simulink model "linetap2"  (Simulink 8.5)
settings: Solver=ode15s  SolverMode=SingleTasking  StartTime=0.0  StopTime=0.1  RelTol=1e-3  AbsTol=1e-3
libraries: powerlib x37
settings Model: Creator=Dr. Lotfifard  LastModifiedBy=PC
settings DataIOCC: LimitDataPoints=off
settings OptimizationCC: BlockReduction=off  BooleanDataType=off
settings DebuggingCC: SaveWithParameterizedLinksMsg=none  SignalResolutionControl=TryResolveAllWithWarning  MultiTaskDSMMsg=warning  MultiTaskCondExecSysMsg=none  FcnCallInpInsideContextMsg=UseLocalSettings  StrictBusMsg=None
settings HardwareCC: TargetUnknown=on

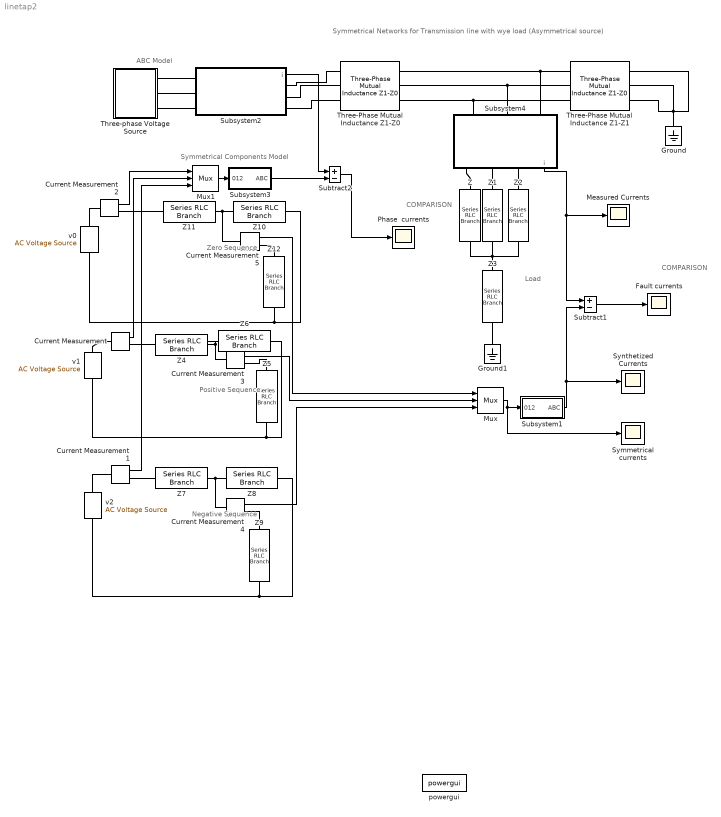
== system linetap2 ==
  note: Symmetrical Networks for Transmission line with wye load (Asymmetrical source)
  note: ABC Model
  note: Symmetrical Components Model
  note: Load
  note: Zero
      | Sequence
  note: Positive
      | Sequence
  note: Negative
      | Sequence
  note: COMPARISON
  note: COMPARISON
  Current Measurement : powerlib/Measurements/Current Measurement  Tag=PoWeRsYsTeMmEaSuReMeNtFiRsT  PhasorSimulation=off  OutputType=Complex  PSBequivalent=0
  Current Measurement{1..5} (5 alike) : powerlib/Measurements/Current Measurement  Tag=PoWeRsYsTeMmEaSuReMeNt  PhasorSimulation=off  OutputType=Complex  PSBequivalent=0
  Fault currents : Scope
      settings: TickLabels=on  TimeRange=0.1  YMin=-3  YMax=3
  Ground : powerlib/Elements/Ground  LConnTagsString=a
  Ground1 : powerlib/Elements/Ground  LConnTagsString=a
  Measured Currents : Scope
      settings: TickLabels=on  TimeRange=0.1  YMin=-3  YMax=3  SaveName=ScopeData2
  Mux : Mux  Inputs=3
  Mux1 : Mux  Inputs=3
  Phase  currents : Scope
      settings: TickLabels=on  TimeRange=0.1  YMin=-23  YMax=23  SaveName=ScopeData3
  Subsystem1 : Subsystem
  Subsystem2 : Subsystem
      mask Display: disp('Current\nMeasurements')
  Subsystem3 : Subsystem
  Subsystem4 : Subsystem
      mask Display: disp('Current\nMeasurements')
  Subtract1 : Sum  Inputs=+-  SaturateOnIntegerOverflow=on  InputSameDT=on  OutDataTypeStr=Inherit: Same as first input
  Subtract2 : Sum  Inputs=+-  SaturateOnIntegerOverflow=on  InputSameDT=on  OutDataTypeStr=Inherit: Same as first input
  Symmetrical currents : Scope
      settings: TickLabels=on  TimeRange=0.05  YMin=-1.05  YMax=1.05  SaveName=ScopeData4
  Synthetized Currents : Scope
      settings: TickLabels=on  TimeRange=0.1  YMin=-3  YMax=3
  Three-Phase Mutual Inductance Z1-Z0 : powerlib/Elements/Three-Phase Mutual Inductance Z1-Z0  LConnTagsString=a|b|c  RConnTagsString=A|B|C  PositiveSequence="[ 0.003  0.015/(2*pi*60)]"  ZeroSequence="[0.006  0.03/(2*pi*60)]"
  Three-Phase Mutual Inductance Z1-Z1 : powerlib/Elements/Three-Phase Mutual Inductance Z1-Z0  LConnTagsString=a|b|c  RConnTagsString=A|B|C  PositiveSequence="[ 0.007  0.035/(2*pi*60)]"  ZeroSequence="[ 0.014  0.07/(2*pi*60)]"
  Three-phase Voltage Source : Subsystem
  Z{,1..2,5,9,12} (6 alike) : powerlib/Elements/Series RLC Branch  LConnTagsString=__new0  RConnTagsString=__new0  BranchType=RL  Resistance=0.72  Inductance=0.54/(2*pi*60)  SetiL0=off  InitialCurrent=0  Capacitance=1e-6  Setx0=off  InitialVoltage=0  Measurements=None
  Z10 : powerlib/Elements/Series RLC Branch  LConnTagsString=__new0  RConnTagsString=__new0  BranchType=RL  Resistance=0.014  Inductance=0.07/(2*pi*60)  SetiL0=off  InitialCurrent=0  Capacitance=1e-6  Setx0=off  InitialVoltage=0  Measurements=None
  Z11 : powerlib/Elements/Series RLC Branch  LConnTagsString=__new0  RConnTagsString=__new0  BranchType=RL  Resistance=0.006  Inductance=0.03/(2*pi*60)  SetiL0=off  InitialCurrent=0  Capacitance=1e-6  Setx0=off  InitialVoltage=0  Measurements=None
  Z3 : powerlib/Elements/Series RLC Branch  LConnTagsString=__new0  RConnTagsString=__new0  BranchType=RL  Resistance=1  Inductance=0  SetiL0=off  InitialCurrent=0  Capacitance=1e-6  Setx0=off  InitialVoltage=0  Measurements=None
  Z4 : powerlib/Elements/Series RLC Branch  LConnTagsString=__new0  RConnTagsString=__new0  BranchType=RL  Resistance=0.003  Inductance=0.015/(2*pi*60)  SetiL0=off  InitialCurrent=0  Capacitance=1e-6  Setx0=off  InitialVoltage=0  Measurements=None
  Z6 : powerlib/Elements/Series RLC Branch  LConnTagsString=__new0  RConnTagsString=__new0  BranchType=RL  Resistance=0.007  Inductance=0.035/(2*pi*60)  SetiL0=off  InitialCurrent=0  Capacitance=1e-6  Setx0=off  InitialVoltage=0  Measurements=None
  Z7 : powerlib/Elements/Series RLC Branch  LConnTagsString=__new0  RConnTagsString=__new0  BranchType=RL  Resistance=0.003  Inductance=0.015/(2*pi*60)  SetiL0=off  InitialCurrent=0  Capacitance=1e-6  Setx0=off  InitialVoltage=0  Measurements=None
  Z8 : powerlib/Elements/Series RLC Branch  LConnTagsString=__new0  RConnTagsString=__new0  BranchType=RL  Resistance=0.007  Inductance=0.035/(2*pi*60)  SetiL0=off  InitialCurrent=0  Capacitance=1e-6  Setx0=off  InitialVoltage=0  Measurements=None
  powergui : powerlib/powergui  SimulationMode=Continuous  SolverType=Tustin/Backward Euler (TBE)  SampleTime=0  frequency=60  SPID=off  DisableSnubberDevices=off  DisableRonSwitches=off  DisableVfSwitches=off  SwTol=0  DisplayEquations=off  Interpol=off  methode=off  Ts=0  FunctionMessages=off  echomessages=off  HookPort=off  EnableUseOfTLC=off  x0status=blocks  frequencyindice=60  Pbase=100e6  ErrMax=1e-4  Iterations=50  UnitsV=kV  UnitsW=MW  buscounter=0  RestoreLinks=warning  ResistiveCurrentMeasurement=off  Frange=[0:2:500]  Ylog=off  Xlog=on  ShowGrid=off  save=off  variable=ZData  structure=0  ZoomFFT=on  StartTime=0.0  cycles=1  DisplayStyle=1  fundamental=60  FreqAxis=off  MaxFrequency=1000  frequencyindicesteady=1  RmsSteady=1  display=off
  v0 : powerlib/Electrical Sources/AC Voltage Source  Amplitude=0.031  Phase=-78  Frequency=60  SampleTime=0  Measurements=None
  v1 : powerlib/Electrical Sources/AC Voltage Source  Amplitude=0.963  Phase=-6.56  Frequency=60  SampleTime=0  Measurements=None
  v2 : powerlib/Electrical Sources/AC Voltage Source  Amplitude=0.145  Phase=75.41  Frequency=60  SampleTime=0  Measurements=None
  wires:
  Mux/1 -> Symmetrical currents/1, Subsystem1/1(012)
  Mux1/1 -> Subsystem3/1(012)
  Current Measurement/1 -> Mux1/2
  Subtract2/1 -> Phase  currents/1
  Current Measurement4/1 -> Mux/3
  Current Measurement3/1 -> Mux/2
  Current Measurement1/1 -> Mux1/3
  Current Measurement2/1 -> Mux1/1
  Current Measurement5/1 -> Mux/1
  Subtract1/1 -> Fault currents/1
  Subsystem1/1(ABC) -> Subtract1/2, Synthetized Currents/1
  Subsystem3/1(ABC) -> Subtract2/2
  Subsystem4/1(i) -> Measured Currents/1, Subtract1/1
  Subsystem2/1(i) -> Subtract2/1
  connections:
  Three-Phase Mutual Inductance Z1-Z1/RConn3 -- Three-Phase Mutual Inductance Z1-Z1/RConn2 -- Ground/LConn1 -- Three-Phase Mutual Inductance Z1-Z1/RConn1
  Z/RConn1 -- Z1/RConn1 -- Z3/LConn1 -- Z2/RConn1
  Subsystem4/LConn1 -- Three-Phase Mutual Inductance Z1-Z0/RConn1 -- Three-Phase Mutual Inductance Z1-Z1/LConn1
  Subsystem4/LConn2 -- Three-Phase Mutual Inductance Z1-Z0/RConn2 -- Three-Phase Mutual Inductance Z1-Z1/LConn2
  Subsystem4/LConn3 -- Three-Phase Mutual Inductance Z1-Z0/RConn3 -- Three-Phase Mutual Inductance Z1-Z1/LConn3
  Z6/LConn1 -- Current Measurement3/LConn1 -- Z4/RConn1
  Z6/RConn1 -- Z5/RConn1 -- v1/LConn1
  Z8/LConn1 -- Z7/RConn1 -- Current Measurement4/LConn1
  v2/LConn1 -- Z8/RConn1 -- Z9/RConn1
  Current Measurement5/LConn1 -- Z10/LConn1 -- Z11/RConn1
  v0/LConn1 -- Z10/RConn1 -- Z12/RConn1
  Z/LConn1 -- Subsystem4/RConn3
  Z2/LConn1 -- Subsystem4/RConn1
  Z1/LConn1 -- Subsystem4/RConn2
  Current Measurement5/RConn1 -- Z12/LConn1
  Current Measurement/RConn1 -- Z4/LConn1
  Z5/LConn1 -- Current Measurement3/RConn1
  Subsystem2/RConn1 -- Three-Phase Mutual Inductance Z1-Z0/LConn1
  Z11/LConn1 -- Current Measurement2/RConn1
  Subsystem2/LConn3 -- Three-phase Voltage Source/RConn3
  Subsystem2/LConn1 -- Three-phase Voltage Source/RConn1
  Three-phase Voltage Source/RConn2 -- Subsystem2/LConn2
  Z3/RConn1 -- Ground1/LConn1
  Current Measurement4/RConn1 -- Z9/LConn1
  Current Measurement2/LConn1 -- v0/RConn1
  Z7/LConn1 -- Current Measurement1/RConn1
  Current Measurement/LConn1 -- v1/RConn1
  Three-Phase Mutual Inductance Z1-Z0/LConn2 -- Subsystem2/RConn2
  Subsystem2/RConn3 -- Three-Phase Mutual Inductance Z1-Z0/LConn3
  Current Measurement1/LConn1 -- v2/RConn1

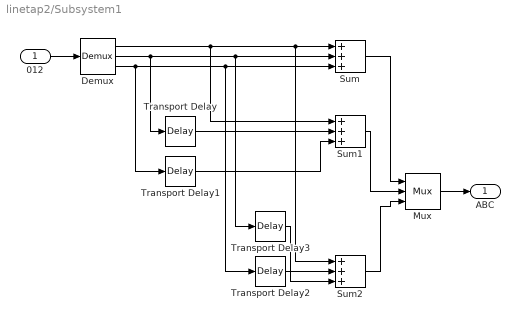
== system linetap2/Subsystem1 ==
  012 : Inport
  Demux : Demux  Outputs=3
  Mux : Mux  Inputs=3
  Sum : Sum  Inputs=+++  SaturateOnIntegerOverflow=on  InputSameDT=on  OutDataTypeStr=Inherit: Same as first input
  Sum1 : Sum  Inputs=+++  SaturateOnIntegerOverflow=on  InputSameDT=on  OutDataTypeStr=Inherit: Same as first input
  Sum2 : Sum  Inputs=+++  SaturateOnIntegerOverflow=on  InputSameDT=on  OutDataTypeStr=Inherit: Same as first input
  Transport Delay : TransportDelay  DelayTime=1/(3*60)
  Transport Delay1 : TransportDelay  DelayTime=2/(3*60)
  Transport Delay2 : TransportDelay  DelayTime=1/(3*60)
  Transport Delay3 : TransportDelay  DelayTime=2/(3*60)
  ABC : Outport  InitialOutput=0
  wires:
  Transport Delay3/1 -> Sum2/2
  Transport Delay2/1 -> Sum2/3
  Transport Delay1/1 -> Sum1/3
  Transport Delay/1 -> Sum1/2
  Demux/1 -> Sum2/1, Sum/1, Sum1/1
  Demux/3 -> Transport Delay2/1, Sum/3, Transport Delay1/1
  Demux/2 -> Transport Delay3/1, Sum/2, Transport Delay/1
  Sum2/1 -> Mux/3
  Mux/1 -> ABC/1
  Sum/1 -> Mux/1
  Sum1/1 -> Mux/2
  012/1 -> Demux/1

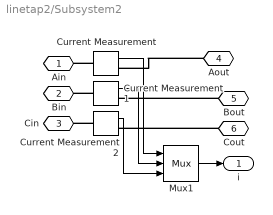
== system linetap2/Subsystem2 ==
  Current Measurement : powerlib/Measurements/Current Measurement  Tag=PoWeRsYsTeMmEaSuReMeNt  PhasorSimulation=off  OutputType=Complex  PSBequivalent=0
  Current Measurement1 : powerlib/Measurements/Current Measurement  Tag=PoWeRsYsTeMmEaSuReMeNt  PhasorSimulation=off  OutputType=Complex  PSBequivalent=0
  Current Measurement2 : powerlib/Measurements/Current Measurement  Tag=PoWeRsYsTeMmEaSuReMeNt  PhasorSimulation=off  OutputType=Complex  PSBequivalent=0
  Mux1 : Mux  Inputs=3
  Ain : PMIOPort  Port=1  Side=Left
  Bin : PMIOPort  Port=2  Side=Left
  Cin : PMIOPort  Port=3  Side=Left
  Aout : PMIOPort  Port=4  Side=Right
  Bout : PMIOPort  Port=5  Side=Right
  Cout : PMIOPort  Port=6  Side=Right
  i : Outport  InitialOutput=0
  wires:
  Current Measurement/1 -> Mux1/1
  Current Measurement1/1 -> Mux1/2
  Current Measurement2/1 -> Mux1/3
  Mux1/1 -> i/1
  connections:
  Cout/RConn1 -- Current Measurement2/RConn1
  Current Measurement2/LConn1 -- Cin/RConn1
  Bout/RConn1 -- Current Measurement1/RConn1
  Current Measurement1/LConn1 -- Bin/RConn1
  Aout/RConn1 -- Current Measurement/RConn1
  Current Measurement/LConn1 -- Ain/RConn1

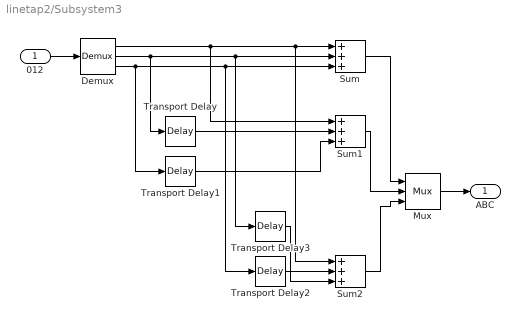
== system linetap2/Subsystem3 ==
  012 : Inport
  Demux : Demux  Outputs=3
  Mux : Mux  Inputs=3
  Sum : Sum  Inputs=+++  SaturateOnIntegerOverflow=on  InputSameDT=on  OutDataTypeStr=Inherit: Same as first input
  Sum1 : Sum  Inputs=+++  SaturateOnIntegerOverflow=on  InputSameDT=on  OutDataTypeStr=Inherit: Same as first input
  Sum2 : Sum  Inputs=+++  SaturateOnIntegerOverflow=on  InputSameDT=on  OutDataTypeStr=Inherit: Same as first input
  Transport Delay : TransportDelay  DelayTime=1/(3*60)
  Transport Delay1 : TransportDelay  DelayTime=2/(3*60)
  Transport Delay2 : TransportDelay  DelayTime=1/(3*60)
  Transport Delay3 : TransportDelay  DelayTime=2/(3*60)
  ABC : Outport  InitialOutput=0
  wires:
  Transport Delay3/1 -> Sum2/2
  Transport Delay2/1 -> Sum2/3
  Transport Delay1/1 -> Sum1/3
  Transport Delay/1 -> Sum1/2
  Demux/1 -> Sum2/1, Sum/1, Sum1/1
  Demux/3 -> Transport Delay2/1, Sum/3, Transport Delay1/1
  Demux/2 -> Transport Delay3/1, Sum/2, Transport Delay/1
  Sum2/1 -> Mux/3
  Mux/1 -> ABC/1
  Sum/1 -> Mux/1
  Sum1/1 -> Mux/2
  012/1 -> Demux/1

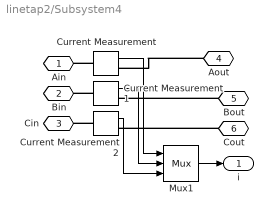
== system linetap2/Subsystem4 ==
  Current Measurement : powerlib/Measurements/Current Measurement  Tag=PoWeRsYsTeMmEaSuReMeNt  PhasorSimulation=off  OutputType=Complex  PSBequivalent=0
  Current Measurement1 : powerlib/Measurements/Current Measurement  Tag=PoWeRsYsTeMmEaSuReMeNt  PhasorSimulation=off  OutputType=Complex  PSBequivalent=0
  Current Measurement2 : powerlib/Measurements/Current Measurement  Tag=PoWeRsYsTeMmEaSuReMeNt  PhasorSimulation=off  OutputType=Complex  PSBequivalent=0
  Mux1 : Mux  Inputs=3
  Ain : PMIOPort  Port=1  Side=Left
  Bin : PMIOPort  Port=2  Side=Left
  Cin : PMIOPort  Port=3  Side=Left
  Aout : PMIOPort  Port=4  Side=Right
  Bout : PMIOPort  Port=5  Side=Right
  Cout : PMIOPort  Port=6  Side=Right
  i : Outport  InitialOutput=0
  wires:
  Current Measurement/1 -> Mux1/1
  Current Measurement1/1 -> Mux1/2
  Current Measurement2/1 -> Mux1/3
  Mux1/1 -> i/1
  connections:
  Cout/RConn1 -- Current Measurement2/RConn1
  Current Measurement2/LConn1 -- Cin/RConn1
  Bout/RConn1 -- Current Measurement1/RConn1
  Current Measurement1/LConn1 -- Bin/RConn1
  Aout/RConn1 -- Current Measurement/RConn1
  Current Measurement/LConn1 -- Ain/RConn1

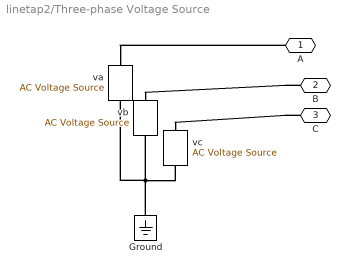
== system linetap2/Three-phase Voltage Source ==
  Ground : powerlib/Elements/Ground  LConnTagsString=a
  va : powerlib/Electrical Sources/AC Voltage Source  Amplitude=1  Phase=0  Frequency=60  SampleTime=0  Measurements=None
  vb : powerlib/Electrical Sources/AC Voltage Source  Amplitude=1.1  Phase=-130  Frequency=60  SampleTime=0  Measurements=None
  vc : powerlib/Electrical Sources/AC Voltage Source  Amplitude=0.8  Phase=110  Frequency=60  SampleTime=0  Measurements=None
  A : PMIOPort  Port=1  Side=Right
  B : PMIOPort  Port=2  Side=Right
  C : PMIOPort  Port=3  Side=Right
  connections:
  Ground/LConn1 -- vb/LConn1 -- vc/LConn1 -- va/LConn1
  A/RConn1 -- va/RConn1
  B/RConn1 -- vb/RConn1
  C/RConn1 -- vc/RConn1
